simulink model "sim2"  (R2022b)
settings: Solver=ode45  StartTime=0.0  StopTime=10.0  MaxStep=0.001  RelTol=1e-6
values from neighbouring files (symbols this model uses):
  cs = 1897.2717254    [quarter_car_parameters.mat]
  ks = 22000    [quarter_car_parameters.mat]
  kt = 176000    [quarter_car_parameters.mat]
  ms = 454.5    [quarter_car_parameters.mat]
  mu = 45.45    [quarter_car_parameters.mat]
  road_case = 4    [quarter_car_parameters.mat]
undefined symbols (not defined in the file or in its folder): active_mode, Fa_max, Kd_pid, Ki_pid, Kp_pid, N_pid
libraries: slpidlib x1
settings Model: Creator=Forough  LastModifiedBy=Forough

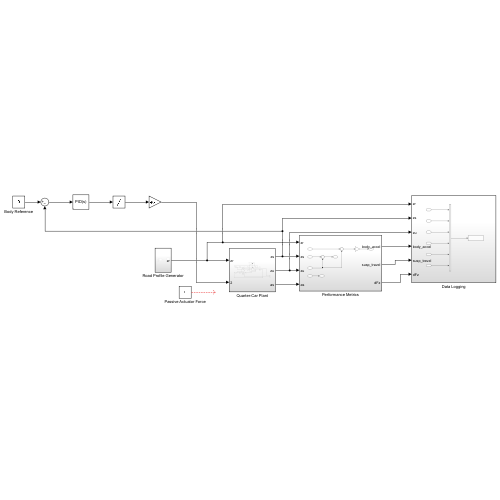
[thumbnail: Simulink's stored preview of the top-level diagram]
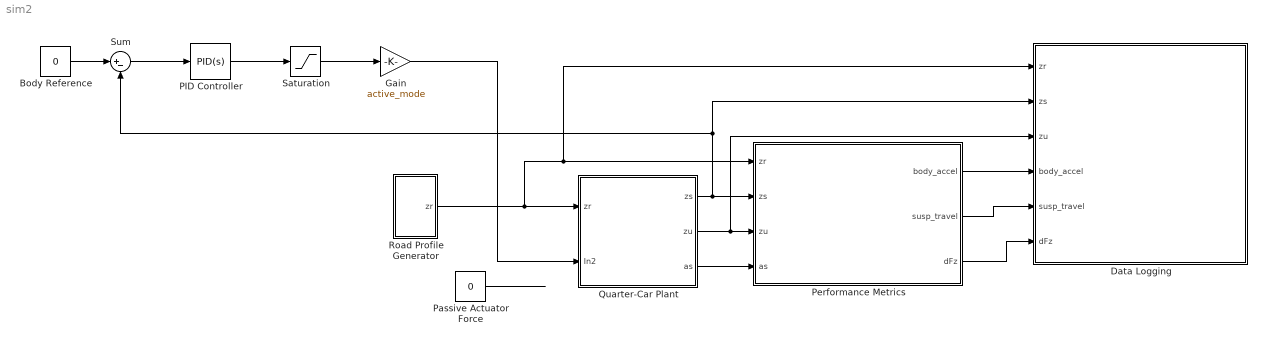
== system sim2 ==
  Body Reference : Constant  Value=0
  Data Logging : Subsystem
  Gain : Gain  Gain=active_mode
  PID Controller : slpidlib/PID Controller  Controller=PID  Form=Parallel  TimeDomain=Continuous-time  UseExternalTs=off  SampleTime=-1  IntegratorMethod=Forward Euler  FilterMethod=Forward Euler  ControllerParametersSource=internal  P=Kp_pid  I=Ki_pid  UseKiTs=off  D=Kd_pid  N=N_pid  UseFilter=on  TunerSelectOption=Transfer Function Based (PID Tuner App)  InitialConditionSource=internal  InitialConditionForIntegrator=0  InitialConditionForFilter=0  DifferentiatorICPrevScaledInput=0  ExternalReset=none  TrackingMode=off  Kt=1  LimitOutput=off  SatLimitsSource=internal  UpperSaturationLimit=inf  LowerSaturationLimit=-inf  LinearizeAsGain=on  AntiWindupMode=none  Kb=1  LimitIntegrator=off  UpperIntegratorSaturationLimit=inf  LowerIntegratorSaturationLimit=-inf  POutMin=[]  POutMax=[]  IOutMin=[]  IOutMax=[]  DOutMin=[]  DOutMax=[]  NOutMin=[]  NOutMax=[]  SumOutMin=[]  SumOutMax=[]  SaturationOutMin=[]  SaturationOutMax=[]  PParamMin=[]  PParamMax=[]  IParamMin=[]  IParamMax=[]  DParamMin=[]  DParamMax=[]  NParamMin=[]  NParamMax=[]  KbParamMin=[]  KbParamMax=[]  KtParamMin=[]  KtParamMax=[]  KbOutMin=[]  KbOutMax=[]  KtOutMin=[]  KtOutMax=[]  IntegratorOutMin=[]  IntegratorOutMax=[]  FilterOutMin=[]  FilterOutMax=[]  SumI1OutMin=[]  SumI1OutMax=[]  SumI2OutMin=[]  SumI2OutMax=[]  SumI3OutMin=[]  SumI3OutMax=[]  SumI4OutMin=[]  SumI4OutMax=[]  SumDOutMin=[]  SumDOutMax=[]  DifferentiatorOutMin=[]  DifferentiatorOutMax=[]  FilterDiffOutCoefMin=[]  FilterDiffOutCoefMax=[]  ReciprocalOutMin=[]  ReciprocalOutMax=[]  SumDenOutMin=[]  SumDenOutMax=[]  SumNumOutMin=[]  SumNumOutMax=[]  DivideOutMin=[]  DivideOutMax=[]  UdiffTsProdOutMin=[]  UdiffTsProdOutMax=[]  NTsProdOutMin=[]  NTsProdOutMax=[]  UintegralTsProdOutMin=[]  UintegralTsProdOutMax=[]  UngainTsProdOutMin=[]  UngainTsProdOutMax=[]  ClampingZeroOutDataTypeStr=Inherit: Inherit via back propagation  ClampingZeroOutMin=[]  ClampingZeroOutMax=[]  FilterDenConstantOutDataTypeStr=Inherit: Inherit via back propagation  FilterDenConstantOutMin=[]  FilterDenConstantOutMax=[]  PCopyOutDataTypeStr=Inherit: Inherit via back propagation  PCopyOutMin=[]  PCopyOutMax=[]  NCopyOutDataTypeStr=Inherit: Inherit via back propagation  NCopyOutMin=[]  NCopyOutMax=[]  IntegratorContinuousStateAttributes=''  IntegratorStateMustResolveToSignalObject=off  IntegratorRTWStateStorageClass=Auto  FilterContinuousStateAttributes=''  FilterStateMustResolveToSignalObject=off  FilterRTWStateStorageClass=Auto  ParallelPVariant=InternalParameters  IdealPVariant=Disabled  IVariant=InternalParameters  DVariant=InternalParameters  IntegratorVariant=Continuous  SatVariant=Disabled  AWVariant=Passthrough  PCopyVariant=Disabled  TRVariant=Disabled  FdbkBlocksVariant=Forward  IdealPFdbkVariant=Disabled  SatFdbkVariant=Disabled  DerivativeFilterVariant=ContFilter  NVariant=InternalParameters  NCopyVariant=Disabled  FilterICVariant=InternalICsFilter  IntegratorICVariant=InternalICs  ExternalResetVariant=Disabled  TRSumVariant=Passthrough  SumFdbkVariant=Disabled  SumVariant=Sum_PID  TsampFilterVariant=InternalTs  TsampNgainVariant=Passthrough  TsampIntegralVariant=Passthrough  ExternalSaturationOutDataTypeStr=Inherit: Same as second input
  Passive Actuator Force : Constant  Value=0
  Performance Metrics : Subsystem
  Quarter-Car Plant : Subsystem
  Road Profile Generator : Subsystem
  Saturation : Saturate  UpperLimit=Fa_max  LowerLimit=-Fa_max
  Sum : Sum  Inputs=|+-
  wires:
  Quarter-Car Plant/1(zs) -> Sum/2, Data Logging/2(zs), Performance Metrics/2(zs)
  Quarter-Car Plant/2(zu) -> Data Logging/3(zu), Performance Metrics/3(zu)
  Quarter-Car Plant/3(as) -> Performance Metrics/4(as)
  Passive Actuator Force/1 -> ?
  Performance Metrics/3(dFz) -> Data Logging/6(dFz)
  Performance Metrics/2(susp_travel) -> Data Logging/5(susp_travel)
  Performance Metrics/1(body_accel) -> Data Logging/4(body_accel)
  Road Profile Generator/1(zr) -> Data Logging/1(zr), Performance Metrics/1(zr), Quarter-Car Plant/1(zr)
  Body Reference/1 -> Sum/1
  Sum/1 -> PID Controller/1
  PID Controller/1 -> Saturation/1
  Saturation/1 -> Gain/1
  Gain/1 -> Quarter-Car Plant/2(In2)

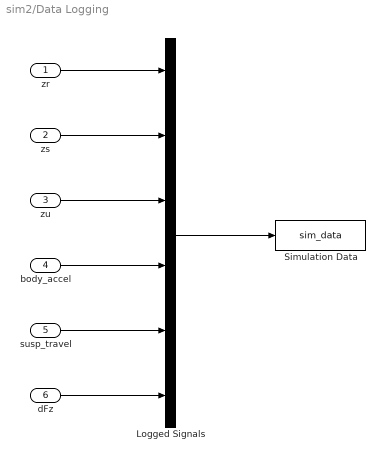
== system sim2/Data Logging ==
  zr : Inport
  zs : Inport  Port=2
  zu : Inport  Port=3
  body_accel : Inport  Port=4
  susp_travel : Inport  Port=5
  dFz : Inport  Port=6
  Logged Signals : Mux  Inputs=6
  Simulation Data : ToWorkspace  VariableName=sim_data  SaveFormat=Timeseries  SampleTime=-1
  wires:
  zr/1 -> Logged Signals/1
  zs/1 -> Logged Signals/2
  zu/1 -> Logged Signals/3
  body_accel/1 -> Logged Signals/4
  susp_travel/1 -> Logged Signals/5
  dFz/1 -> Logged Signals/6
  Logged Signals/1 -> Simulation Data/1

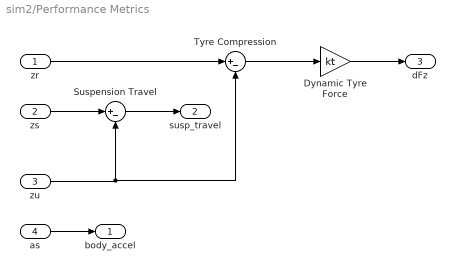
== system sim2/Performance Metrics ==
  zr : Inport
  zs : Inport  Port=2
  zu : Inport  Port=3
  as : Inport  Port=4
  Dynamic Tyre Force : Gain  Gain=kt
  Suspension Travel : Sum  Inputs=|+-
  Tyre Compression : Sum  Inputs=|+-
  body_accel : Outport
  susp_travel : Outport  Port=2
  dFz : Outport  Port=3
  wires:
  as/1 -> body_accel/1
  zs/1 -> Suspension Travel/1
  zu/1 -> Tyre Compression/2, Suspension Travel/2
  zr/1 -> Tyre Compression/1
  Tyre Compression/1 -> Dynamic Tyre Force/1
  Dynamic Tyre Force/1 -> dFz/1
  Suspension Travel/1 -> susp_travel/1

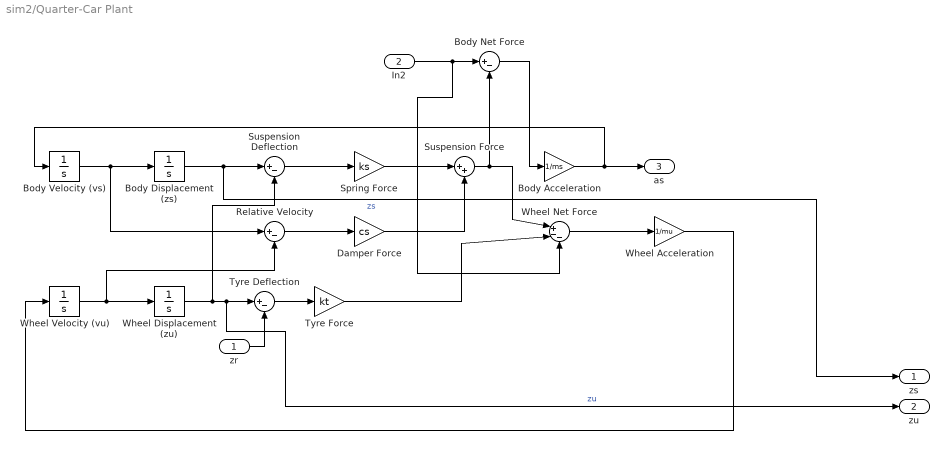
== system sim2/Quarter-Car Plant ==
  zr : Inport
  In2 : Inport  Port=2
  Body Acceleration : Gain  Gain=1/ms
  Body Displacement (zs) : Integrator
  Body Net Force : Sum  Inputs=|+-
  "Body Velocity (vs) " : Integrator
  Damper Force : Gain  Gain=cs
  Relative Velocity : Sum  Inputs=|+-
  Spring Force : Gain  Gain=ks
  Suspension Deflection : Sum  Inputs=|+-
  Suspension Force : Sum  Inputs=|++
  Tyre Deflection : Sum  Inputs=|+-
  Tyre Force : Gain  Gain=kt
  Wheel Acceleration : Gain  Gain=1/mu
  Wheel Displacement (zu) : Integrator
  Wheel Net Force : Sum  Inputs=|+--
  "Wheel Velocity (vu) " : Integrator
  zs : Outport
  zu : Outport  Port=2
  as : Outport  Port=3
  wires:
  Relative Velocity/1 -> Damper Force/1
  Wheel Displacement (zu)/1 -> zu/1, Tyre Deflection/1, Suspension Deflection/2  "zu"
  "Wheel Velocity (vu) "/1 -> Relative Velocity/2, Wheel Displacement (zu)/1
  Body Displacement (zs)/1 -> zs/1, Suspension Deflection/1  "zs"
  Suspension Force/1 -> Wheel Net Force/1, Body Net Force/2
  Damper Force/1 -> Suspension Force/2
  "Body Velocity (vs) "/1 -> Relative Velocity/1, Body Displacement (zs)/1
  Tyre Deflection/1 -> Tyre Force/1
  Body Acceleration/1 -> as/1, "Body Velocity (vs) "/1
  Wheel Acceleration/1 -> "Wheel Velocity (vu) "/1
  Suspension Deflection/1 -> Spring Force/1
  Wheel Net Force/1 -> Wheel Acceleration/1
  Spring Force/1 -> Suspension Force/1
  Tyre Force/1 -> Wheel Net Force/2
  zr/1 -> Tyre Deflection/2
  In2/1 -> Wheel Net Force/3, Body Net Force/1
  Body Net Force/1 -> Body Acceleration/1

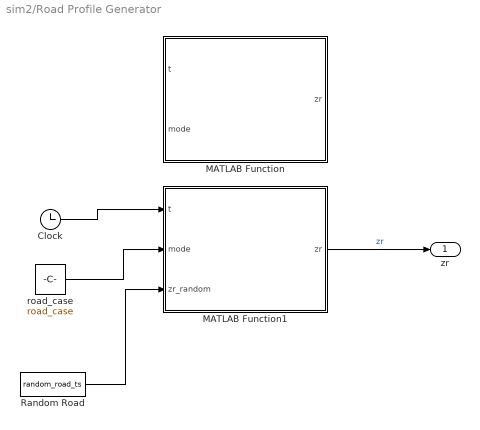
== system sim2/Road Profile Generator ==
  Clock : Clock
  MATLAB Function : MATLAB Function  TreatAsAtomicUnit=on
  MATLAB Function1 : MATLAB Function  TreatAsAtomicUnit=on
  Random Road : FromWorkspace  VariableName=random_road_ts  OutputAfterFinalValue=Holding final value
  road_case : Constant  Value=road_case
  zr : Outport
  wires:
  MATLAB Function1/1(zr) -> zr/1  "zr"
  Clock/1 -> MATLAB Function1/1(t)
  road_case/1 -> MATLAB Function1/2(mode)
  Random Road/1 -> MATLAB Function1/3(zr_random)

== matlab function sim2/Road Profile Generator/MATLAB Function ==
  data: t input; zr output; mode input
function zr = road_profile(t, mode)

switch mode
    case 1
        h = 0.05;
        t0 = 1;
        zr = h*(t >= t0);

    case 2
        h = 0.05;
        t0 = 1;
        L = 3;
        V = 10;
        T = L/V;

        if t >= t0 && t <= t0 + T
            tau = t - t0;
            zr = 0.5*h*(1 - cos(2*pi*tau/T));
        else
            zr = 0;
        end

    case 3
        A = 0.02;
        f = 1.5;
        t0 = 1;

        if t >= t0
            zr = A*sin(2*pi*f*(t - t0));
        else
            zr = 0;
        end

    otherwise
        zr = 0;
end

== matlab function sim2/Road Profile Generator/MATLAB Function1 ==
  data: t input; zr output; mode input; zr_random input
function zr = road_profile(t, mode, zr_random)

switch mode
    case 1
        h = 0.05;
        t0 = 1;
        zr = h*(t >= t0);

    case 2
        h = 0.05;
        t0 = 1;
        L = 3;
        V = 10;
        T = L/V;

        if t >= t0 && t <= t0 + T
            tau = t - t0;
            zr = 0.5*h*(1 - cos(2*pi*tau/T));
        else
            zr = 0;
        end

    case 3
        A = 0.02;
        f = 1.5;
        t0 = 1;

        if t >= t0
            zr = A*sin(2*pi*f*(t - t0));
        else
            zr = 0;
        end

    case 4
        zr = zr_random;

    otherwise
        zr = 0;
end
